simulink model "bat_inv_psm"  (R2025b)
settings: Solver=ode1be  StartTime=0.0  StopTime=simlength  FixedStep=tc  MaxStep=tc
undefined symbols (not defined in the file): b, CTRPIFF_CLIP_RELEASE, dead_time_INV, dead_time_STEPUP, emf_fb_p, emf_fb_p_ccaller_1, emf_fb_p_ccaller_2, emf_p, emf_p_ccaller_1, emf_p_ccaller_2, fPWM_INV, fPWM_STEPUP, g0_161Hz, g1_161Hz, i_grid_neg_eta_lim, i_grid_neg_eta_red_lim, i_grid_neg_xi_lim, i_grid_neg_xi_red_lim, i_grid_pos_eta_lim, i_grid_pos_eta_red_lim, ibez, id_lim, idc_bez, iq_lim, Jm, k_frt_ref, kg, ki_i, ki_ib, ki_vs, ki_w, kp_i, kp_ib, kp_vs, kp_w, kw, l1, l2, Lb, Ld_norm, Lq_norm, Ls_norm, magnitude, motorc_m_scale, number_of_cells, omega_bez, omega_m_bez, omega_m_sim, psi_bez, psi_m, psi_m_norm, Q, q1Kalman, q2Kalman, q3Kalman, rKalman, RLb, rpm_bez, rpm_sim, rpm_torque_curve ... (+17)
libraries: fl_lib x87, nesl_utility x66, simulink x4, singlephase_inductor_with_saturation_lib x2, threephase_inductor_lib x1, ee_lib x1, lithium_ion_cell_lib x1, flexshaft_lib x1, pmsm_uvw_with_harmonics_lib x1
(part 3 of 5)

== system bat_inv_psm/afe_abc_inv_psm_mod1/stepup/switch_2 ==
  Diode : fl_lib/Electrical/Electrical Elements/Diode  Vf=Vgamma V  Ron=Ron Ohm  Goff=1e-8 1/Ohm  i_specify=off  i_priority=None  i=0 A  i_nominal_specify=off  i_nominal_value=1  i_nominal_unit=A  v_specify=off  v_priority=None  v=0 V  v_nominal_specify=off  v_nominal_value=1  v_nominal_unit=V
  Switch : fl_lib/Electrical/Electrical Elements/Switch  R_closed=Ron Ohm  G_open=1e-8 1/Ohm  Threshold=7.5  i_specify=off  i_priority=None  i=0 A  i_nominal_specify=off  i_nominal_value=1  i_nominal_unit=A  v_specify=off  v_priority=None  v=0 V  v_nominal_specify=off  v_nominal_value=1  v_nominal_unit=V
  snubber : fl_lib/Electrical/Electrical Elements/Capacitor  c=Csnubber F  r=Rsnubber Ohm  g=0 1/Ohm  i_specify=off  i_priority=None  i=0 A  i_nominal_specify=off  i_nominal_value=1  i_nominal_unit=A  v_specify=off  v_priority=None  v=0 V  v_nominal_specify=off  v_nominal_value=1  v_nominal_unit=V  vc_specify=off  vc_priority=High  vc=0 V  vc_nominal_specify=off  vc_nominal_value=1  vc_nominal_unit=V
  G : PMIOPort  Side=Left
  C : PMIOPort  Port=2  Side=Left
  E : PMIOPort  Port=3  Side=Right
  connections:
  Switch/RConn2 -- C/RConn1 -- snubber/LConn1 -- Diode/RConn1
  Switch/RConn1 -- G/RConn1
  Switch/LConn1 -- E/RConn1 -- snubber/RConn1 -- Diode/LConn1

== system bat_inv_psm/afe_abc_inv_psm_mod1/stepup_control/idc_ctrl ==
  idc_pu : Inport
  idc_pu_ref : Inport  Port=2
  1/Ti : Gain  Gain=kp_ib  SaturateOnIntegerOverflow=on  OutDataTypeStr=Inherit: Same as input  ParamDataTypeStr=Inherit: Same as input
  Gain : Gain
  Saturation : Saturate  UpperLimit=1  LowerLimit=0
  Sum1 : Sum  Inputs=+++  SaturateOnIntegerOverflow=on
  Sum2 : Sum  Inputs=-+  SaturateOnIntegerOverflow=on
  Sum3 : Sum  Inputs=-+  SaturateOnIntegerOverflow=on
  Unit Delay1 : UnitDelay  SampleTime=ts_stepup  HasFrameUpgradeWarning=on
  Unit Delay4 : UnitDelay  SampleTime=ts_stepup  HasFrameUpgradeWarning=on
  kp : Gain  Gain=ki_ib*ts_stepup  SaturateOnIntegerOverflow=on  OutDataTypeStr=Inherit: Same as input  ParamDataTypeStr=Inherit: Same as input
  m_stepup : Outport
  wires:
  Gain/1 -> Unit Delay1/1
  Saturation/1 -> Sum3/2, Gain/1
  Sum1/1 -> Saturation/1
  Sum2/1 -> 1/Ti/1, kp/1
  idc_pu/1 -> Sum2/1
  idc_pu_ref/1 -> Sum2/2
  Unit Delay4/1 -> Sum1/3
  Sum3/1 -> Unit Delay4/1
  kp/1 -> Sum1/2
  1/Ti/1 -> Sum3/1, Sum1/1
  Unit Delay1/1 -> m_stepup/1

== system bat_inv_psm/afe_abc_inv_psm_mod1/stepup_control/udc_ctrl ==
  udc_pu : Inport
  udc_pu_ref : Inport  Port=2
  1/Ti : Gain  Gain=kp_vs  SaturateOnIntegerOverflow=on  OutDataTypeStr=Inherit: Same as input  ParamDataTypeStr=Inherit: Same as input
  Gain : Gain
  Saturation : Saturate  UpperLimit=1.4  LowerLimit=-1.4
  Sum1 : Sum  Inputs=+++  SaturateOnIntegerOverflow=on
  Sum2 : Sum  Inputs=-+  SaturateOnIntegerOverflow=on
  Sum3 : Sum  Inputs=-+  SaturateOnIntegerOverflow=on
  Unit Delay4 : UnitDelay  SampleTime=ts_stepup  HasFrameUpgradeWarning=on
  kp : Gain  Gain=ki_vs*ts_stepup  SaturateOnIntegerOverflow=on  OutDataTypeStr=Inherit: Same as input  ParamDataTypeStr=Inherit: Same as input
  idc_ref : Outport
  wires:
  1/Ti/1 -> Sum3/1, Sum1/1
  kp/1 -> Sum1/2
  Sum3/1 -> Unit Delay4/1
  Unit Delay4/1 -> Sum1/3
  udc_pu_ref/1 -> Sum2/2
  udc_pu/1 -> Sum2/1
  Sum2/1 -> kp/1, 1/Ti/1
  Sum1/1 -> Saturation/1
  Saturation/1 -> Sum3/2, Gain/1
  Gain/1 -> idc_ref/1

== system bat_inv_psm/battery/battery_system/LithiumIonBattery ==
  Current Sensor : fl_lib/Electrical/Electrical Sensors/Current Sensor
  Electrical Reference1 : fl_lib/Electrical/Electrical Elements/Electrical Reference
  PS-Simulink Converter4 : nesl_utility/PS-Simulink Converter  PhysicalDomain=network_engine_domain  SubClassName=ps_output  LeftPortType=input  RightPortType=output  PseudoPeriodic=off  Frequencies=[]  VectorFormat=1-D array  Unit=1  AffineConversion=off
  PS-Simulink Converter5 : nesl_utility/PS-Simulink Converter  PhysicalDomain=network_engine_domain  SubClassName=ps_output  LeftPortType=input  RightPortType=output  PseudoPeriodic=off  Frequencies=[]  VectorFormat=1-D array  Unit=V  AffineConversion=on
  SOC_estimator : Subsystem  Commented=on
  To Workspace1 : ToWorkspace  VariableName=idc_battery_sim  SampleTime=tc
      settings: MaxDataPoints=Nc
  To Workspace2 : ToWorkspace  VariableName=udc_battery_sim  SampleTime=tc
      settings: MaxDataPoints=Nc
  Unit Delay5 : UnitDelay  SampleTime=ts_stepup  HasFrameUpgradeWarning=on
  Voltage Sensor : fl_lib/Electrical/Electrical Sensors/Voltage Sensor
  ibat/vdc : Scope  NumInputPorts=2
      settings: SampleTime=tc  ActiveDisplayYMinimum=-1320.0904644876443  ActiveDisplayYMaximum=5476.2315205150016  DataLoggingVariableName=ScopeData6
  lithium ion cell analytical ocv : Subsystem
  Uout+ : PMIOPort  Side=Right
  Uout- : PMIOPort  Port=2  Side=Right
  wires:
  PS-Simulink Converter5/1 -> Unit Delay5/1
  PS-Simulink Converter4/1 -> To Workspace1/1, ibat/vdc/1  "i batt"
  Unit Delay5/1 -> To Workspace2/1, [vdc]
  [vdc] -> ibat/vdc/2  "vdc"
  connections:
  Current Sensor/RConn1 -- PS-Simulink Converter4/LConn1
  Uout+/RConn1 -- Current Sensor/RConn2 -- Voltage Sensor/LConn1
  Voltage Sensor/RConn1 -- PS-Simulink Converter5/LConn1
  Voltage Sensor/RConn2 -- Electrical Reference1/LConn1 -- lithium ion cell analytical ocv/RConn2 -- Uout-/RConn1
  lithium ion cell analytical ocv/RConn1 -- Current Sensor/LConn1

== system bat_inv_psm/afe_abc_inv_psm_mod1/inverter/inverter/sv_pwm ==
  ab : Inport
  enable : Inport  Port=2
  Bus Selector : BusSelector  OutputSignals=da,db,dc
  Bus Selector1 : BusSelector  OutputSignals=ua,ub
  C Caller : CCaller  FunctionName=sv_pwm_process_simulink  PortSpecificationStruct="%)30     .    V @   8    (     @         %    \"     4    !     0         %  0 \"0    $    _    07)G3F%M90  4&]R=$YA;64 4V-O<&4     26YD97@     5'EP90      4VEZ90      27-';&]B86P   X    P    !@    @    $          4    (     0    ,    !         !   P!O=70 #@   #     &    \"     0         !0    @    !     P    $         $  # &]U=  .    .     8    (    !          %    \"     $    &     0         0   ...(+2669 chars)"  SampleTime=ts_inv
  Constant : Constant  Value=ts_inv
  Data Type Conversion1 : DataTypeConversion  OutDataTypeStr=double  SaturateOnIntegerOverflow=off  RndMeth=Floor
  Data Type Conversion15 : DataTypeConversion  OutDataTypeStr=single  SaturateOnIntegerOverflow=off  RndMeth=Floor
  Data Type Conversion16 : DataTypeConversion  OutDataTypeStr=single  SaturateOnIntegerOverflow=off  RndMeth=Floor
  Data Type Conversion17 : DataTypeConversion  OutDataTypeStr=uint32  SaturateOnIntegerOverflow=off  RndMeth=Floor
  Data Type Conversion18 : DataTypeConversion  OutDataTypeStr=single  SaturateOnIntegerOverflow=off  RndMeth=Floor
  Data Type Conversion2 : DataTypeConversion  OutDataTypeStr=double  SaturateOnIntegerOverflow=off  RndMeth=Floor
  Data Type Conversion3 : DataTypeConversion  OutDataTypeStr=double  SaturateOnIntegerOverflow=off  RndMeth=Floor
  Zero-Order Hold{,1..3} (4 alike) : ZeroOrderHold  SampleTime=ts_afe
  modulator1 : Subsystem
  firing_gates : Outport
  wires:
  Data Type Conversion1/1 -> modulator1/1(u)  "du"
  Zero-Order Hold/1 -> C Caller/1
  Zero-Order Hold2/1 -> C Caller/3
  Constant/1 -> Data Type Conversion16/1
  Data Type Conversion18/1 -> Zero-Order Hold/1
  enable/1 -> Data Type Conversion17/1
  Data Type Conversion2/1 -> modulator1/2(v)  "dv"
  Data Type Conversion16/1 -> Zero-Order Hold2/1
  Zero-Order Hold1/1 -> C Caller/2
  Data Type Conversion17/1 -> Zero-Order Hold3/1
  Zero-Order Hold3/1 -> C Caller/4
  Data Type Conversion15/1 -> Zero-Order Hold1/1
  C Caller/1 -> Bus Selector/1  "out"
  Data Type Conversion3/1 -> modulator1/3(w)  "dw"
  modulator1/1(cmd_gates) -> firing_gates/1
  ab/1 -> Bus Selector1/1
  Bus Selector1/1 -> Data Type Conversion18/1  "<ua>"
  Bus Selector1/2 -> Data Type Conversion15/1  "<ub>"
  Bus Selector/1 -> Data Type Conversion1/1  "<da>"
  Bus Selector/3 -> Data Type Conversion3/1  "<dc>"
  Bus Selector/2 -> Data Type Conversion2/1  "<db>"

== system bat_inv_psm/afe_abc_inv_psm_mod1/inverter/inverter/switch_1 ==
  Diode : fl_lib/Electrical/Electrical Elements/Diode  Vf=Vgamma V  Ron=Ron Ohm  Goff=1e-8 1/Ohm  i_specify=off  i_priority=None  i=0 A  i_nominal_specify=off  i_nominal_value=1  i_nominal_unit=A  v_specify=off  v_priority=None  v=0 V  v_nominal_specify=off  v_nominal_value=1  v_nominal_unit=V
  Switch : fl_lib/Electrical/Electrical Elements/Switch  R_closed=Ron Ohm  G_open=1e-8 1/Ohm  Threshold=7.5  i_specify=off  i_priority=None  i=0 A  i_nominal_specify=off  i_nominal_value=1  i_nominal_unit=A  v_specify=off  v_priority=None  v=0 V  v_nominal_specify=off  v_nominal_value=1  v_nominal_unit=V
  G : PMIOPort  Side=Left
  C : PMIOPort  Port=2  Side=Left
  E : PMIOPort  Port=3  Side=Right
  connections:
  Switch/RConn2 -- C/RConn1 -- Diode/RConn1
  Switch/RConn1 -- G/RConn1
  Switch/LConn1 -- E/RConn1 -- Diode/LConn1

== system bat_inv_psm/afe_abc_inv_psm_mod1/inverter/inverter/switch_2 ==
  Diode : fl_lib/Electrical/Electrical Elements/Diode  Vf=Vgamma V  Ron=Ron Ohm  Goff=1e-8 1/Ohm  i_specify=off  i_priority=None  i=0 A  i_nominal_specify=off  i_nominal_value=1  i_nominal_unit=A  v_specify=off  v_priority=None  v=0 V  v_nominal_specify=off  v_nominal_value=1  v_nominal_unit=V
  Switch : fl_lib/Electrical/Electrical Elements/Switch  R_closed=Ron Ohm  G_open=1e-8 1/Ohm  Threshold=7.5  i_specify=off  i_priority=None  i=0 A  i_nominal_specify=off  i_nominal_value=1  i_nominal_unit=A  v_specify=off  v_priority=None  v=0 V  v_nominal_specify=off  v_nominal_value=1  v_nominal_unit=V
  G : PMIOPort  Side=Left
  C : PMIOPort  Port=2  Side=Left
  E : PMIOPort  Port=3  Side=Right
  connections:
  Diode/LConn1 -- E/RConn1 -- Switch/LConn1
  Switch/RConn1 -- G/RConn1
  Diode/RConn1 -- C/RConn1 -- Switch/RConn2

== system bat_inv_psm/afe_abc_inv_psm_mod1/inverter/inverter/switch_3 ==
  Diode : fl_lib/Electrical/Electrical Elements/Diode  Vf=Vgamma V  Ron=Ron Ohm  Goff=1e-8 1/Ohm  i_specify=off  i_priority=None  i=0 A  i_nominal_specify=off  i_nominal_value=1  i_nominal_unit=A  v_specify=off  v_priority=None  v=0 V  v_nominal_specify=off  v_nominal_value=1  v_nominal_unit=V
  Switch : fl_lib/Electrical/Electrical Elements/Switch  R_closed=Ron Ohm  G_open=1e-8 1/Ohm  Threshold=7.5  i_specify=off  i_priority=None  i=0 A  i_nominal_specify=off  i_nominal_value=1  i_nominal_unit=A  v_specify=off  v_priority=None  v=0 V  v_nominal_specify=off  v_nominal_value=1  v_nominal_unit=V
  G : PMIOPort  Side=Left
  C : PMIOPort  Port=2  Side=Left
  E : PMIOPort  Port=3  Side=Right
  connections:
  Diode/LConn1 -- E/RConn1 -- Switch/LConn1
  Switch/RConn1 -- G/RConn1
  Diode/RConn1 -- C/RConn1 -- Switch/RConn2

== system bat_inv_psm/afe_abc_inv_psm_mod1/inverter/inverter/switch_4 ==
  Diode : fl_lib/Electrical/Electrical Elements/Diode  Vf=Vgamma V  Ron=Ron Ohm  Goff=1e-8 1/Ohm  i_specify=off  i_priority=None  i=0 A  i_nominal_specify=off  i_nominal_value=1  i_nominal_unit=A  v_specify=off  v_priority=None  v=0 V  v_nominal_specify=off  v_nominal_value=1  v_nominal_unit=V
  Switch : fl_lib/Electrical/Electrical Elements/Switch  R_closed=Ron Ohm  G_open=1e-8 1/Ohm  Threshold=7.5  i_specify=off  i_priority=None  i=0 A  i_nominal_specify=off  i_nominal_value=1  i_nominal_unit=A  v_specify=off  v_priority=None  v=0 V  v_nominal_specify=off  v_nominal_value=1  v_nominal_unit=V
  G : PMIOPort  Side=Left
  C : PMIOPort  Port=2  Side=Left
  E : PMIOPort  Port=3  Side=Right
  connections:
  Switch/RConn2 -- C/RConn1 -- Diode/RConn1
  Switch/RConn1 -- G/RConn1
  Switch/LConn1 -- E/RConn1 -- Diode/LConn1

== system bat_inv_psm/afe_abc_inv_psm_mod1/inverter/inverter/switch_5 ==
  Diode : fl_lib/Electrical/Electrical Elements/Diode  Vf=Vgamma V  Ron=Ron Ohm  Goff=1e-8 1/Ohm  i_specify=off  i_priority=None  i=0 A  i_nominal_specify=off  i_nominal_value=1  i_nominal_unit=A  v_specify=off  v_priority=None  v=0 V  v_nominal_specify=off  v_nominal_value=1  v_nominal_unit=V
  Switch : fl_lib/Electrical/Electrical Elements/Switch  R_closed=Ron Ohm  G_open=1e-8 1/Ohm  Threshold=7.5  i_specify=off  i_priority=None  i=0 A  i_nominal_specify=off  i_nominal_value=1  i_nominal_unit=A  v_specify=off  v_priority=None  v=0 V  v_nominal_specify=off  v_nominal_value=1  v_nominal_unit=V
  G : PMIOPort  Side=Left
  C : PMIOPort  Port=2  Side=Left
  E : PMIOPort  Port=3  Side=Right
  connections:
  Diode/LConn1 -- E/RConn1 -- Switch/LConn1
  Switch/RConn1 -- G/RConn1
  Diode/RConn1 -- C/RConn1 -- Switch/RConn2

== system bat_inv_psm/afe_abc_inv_psm_mod1/inverter/inverter/switch_6 ==
  Diode : fl_lib/Electrical/Electrical Elements/Diode  Vf=Vgamma V  Ron=Ron Ohm  Goff=1e-8 1/Ohm  i_specify=off  i_priority=None  i=0 A  i_nominal_specify=off  i_nominal_value=1  i_nominal_unit=A  v_specify=off  v_priority=None  v=0 V  v_nominal_specify=off  v_nominal_value=1  v_nominal_unit=V
  Switch : fl_lib/Electrical/Electrical Elements/Switch  R_closed=Ron Ohm  G_open=1e-8 1/Ohm  Threshold=7.5  i_specify=off  i_priority=None  i=0 A  i_nominal_specify=off  i_nominal_value=1  i_nominal_unit=A  v_specify=off  v_priority=None  v=0 V  v_nominal_specify=off  v_nominal_value=1  v_nominal_unit=V
  G : PMIOPort  Side=Left
  C : PMIOPort  Port=2  Side=Left
  E : PMIOPort  Port=3  Side=Right
  connections:
  Switch/RConn2 -- C/RConn1 -- Diode/RConn1
  Switch/RConn1 -- G/RConn1
  Switch/LConn1 -- E/RConn1 -- Diode/LConn1

== system bat_inv_psm/afe_abc_inv_psm_mod1/inverter_control/current_ctrl/bemf_observer ==
  ialpha_pu : Inport
  ibeta_pu : Inport  Port=2
  ualpha_pu : Inport  Port=3
  ubeta_pu : Inport  Port=4
  BEMF Observer simulink/Ccaller : Scope  NumInputPorts=2
      settings: SampleTime=tc  ActiveDisplayYMinimum=-1.2577905803918839  ActiveDisplayYMaximum=1.2568866163492203
  Mux : Mux  Inputs=3
  Mux1 : Mux  Inputs=3
  Variant Source : VariantSource  VariantControls={use_observer_from_simulink_module_1 == 1, use_observer_from_ccaller_module_1 == 1}
  Variant Source1 : VariantSource  VariantControls={use_observer_from_simulink_module_1 == 1, use_observer_from_ccaller_module_1 == 1}
  bemf_observer : Subsystem
  bemf_observer_ccaller : Subsystem
  double_integrator_observer : Subsystem
  phase_fault : Subsystem
  tag scope: omega_hat_pu=global, theta_hat=global
  wires:
  ialpha_pu/1 -> bemf_observer/1(ialpha_pu), bemf_observer_ccaller/1(ialpha_pu)
  ibeta_pu/1 -> bemf_observer/2(ibeta_pu), bemf_observer_ccaller/2(ibeta_pu)
  Mux/1 -> BEMF Observer simulink/Ccaller/1
  Mux1/1 -> BEMF Observer simulink/Ccaller/2
  double_integrator_observer/1(omega_pu_hat) -> Mux/3  "omega_pu_encoder"
  ualpha_pu/1 -> bemf_observer/3(ualpha_pu), bemf_observer_ccaller/3(ualpha_pu)
  ubeta_pu/1 -> bemf_observer/4(ubeta_pu), bemf_observer_ccaller/4(ubeta_pu)
  double_integrator_observer/2(theta_hat) -> Mux1/3  "theta_hat_encoder"
  [theta_elec_pmsm] -> phase_fault/1(theta_pmsm)  "theta_pmsm"
  phase_fault/1(theta) -> double_integrator_observer/1(theta)
  bemf_observer/1(omega_pu) -> Mux/1, Variant Source/1  "omega_pu"
  bemf_observer_ccaller/2(theta_hat) -> Mux1/2, Variant Source1/2  "theta_hat_code"
  bemf_observer_ccaller/1(omega_pu) -> Mux/2, Variant Source/2  "omega_pu_code"
  bemf_observer/2(theta_hat) -> Variant Source1/1, Mux1/1  "theta_hat"
  Variant Source1/1 -> [theta_hat]
  Variant Source/1 -> [omega_hat_pu]

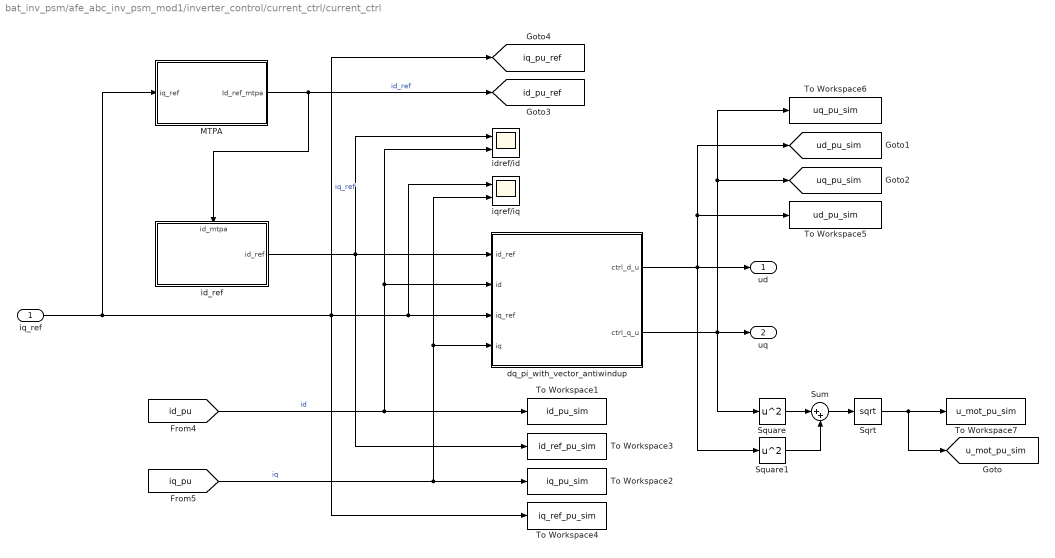
== system bat_inv_psm/afe_abc_inv_psm_mod1/inverter_control/current_ctrl/current_ctrl ==
  iq_ref : Inport
  MTPA : Subsystem
  Sqrt : Sqrt
  Square : Math  Operator=square
  Square1 : Math  Operator=square
  Sum : Sum  Inputs=|++
  To Workspace1 : ToWorkspace  VariableName=id_pu_sim  SampleTime=ts_inv
      settings: MaxDataPoints=Ns_inv
  To Workspace2 : ToWorkspace  VariableName=iq_pu_sim  SampleTime=ts_inv
      settings: MaxDataPoints=Ns_inv
  To Workspace3 : ToWorkspace  VariableName=id_ref_pu_sim  SampleTime=ts_inv
      settings: MaxDataPoints=Ns_inv
  To Workspace4 : ToWorkspace  VariableName=iq_ref_pu_sim  SampleTime=ts_inv
      settings: MaxDataPoints=Ns_inv
  To Workspace5 : ToWorkspace  VariableName=ud_pu_sim  SampleTime=ts_inv
      settings: MaxDataPoints=Ns_inv
  To Workspace6 : ToWorkspace  VariableName=uq_pu_sim  SampleTime=ts_inv
      settings: MaxDataPoints=Ns_inv
  To Workspace7 : ToWorkspace  VariableName=u_mot_pu_sim  SampleTime=ts_inv
      settings: MaxDataPoints=Ns_inv
  dq_pi_with_vector_antiwindup : Subsystem
  id_ref : Subsystem
      settings: PortSchema="{\"entries\":[{\"content\":{\"sides\":[{\"content\":{},\"type\":\"ConnectorPlacement.EquallySpacedRectSide\",\"uuid\":\"42af5d69-f0eb-42c6-9e03-28c1d0757323\"},{\"content\":{\"connectorIds\":[\"Out1\"],\"side\":\"RIGHT\"},\"type\":\"ConnectorPlacement.EquallySpacedRectSide\",\"uuid\":\"dd68a9f9-d15f-4e57-9d9e-130889a7b90c\"},{\"content\":{\"connectorIds\":[\"In1\"],\"side\":\"TOP\"},\"type\":\"ConnectorPlacement.EquallySpacedRectSide\",\"uuid\":\"68c797a2-8439-4b8d-8368-b7485adf0676\"}]},\"type\":\"ConnectorPlacement.EquallySpacedConnector\",\"uuid\":\"693c5f1c-0580-4626-8f13-b27865dfb3ac\"}],\"packageUris\":[\"http://schema.mathworks.com/mf0/Connector/R2020b\"],\"version\":\"1.0\"}"
  idref/id : Scope  NumInputPorts=2
      settings: SampleTime=tc  ActiveDisplayYMinimum=-0.5383825399353187  ActiveDisplayYMaximum=0.059820282309629005
  iqref/iq : Scope  NumInputPorts=2
      settings: SampleTime=tc  ActiveDisplayYMinimum=-1.1641617765003931  ActiveDisplayYMaximum=0.12935130850004364  DataLoggingVariableName=ScopeData2
  ud : Outport
  uq : Outport  Port=2
  tag scope: id_pu_ref=global, iq_pu_ref=global, u_mot_pu_sim=global, ud_pu_sim=global, uq_pu_sim=global
  wires:
  [iq_pu] -> To Workspace2/1, iqref/iq/2, dq_pi_with_vector_antiwindup/4(iq)  "iq"
  [id_pu] -> To Workspace1/1, idref/id/2, dq_pi_with_vector_antiwindup/2(id)  "id"
  MTPA/1(Id_ref_mtpa) -> id_ref/1(id_mtpa), [id_pu_ref]  "id_ref"
  iq_ref/1 -> MTPA/1(iq_ref), To Workspace4/1, iqref/iq/1, dq_pi_with_vector_antiwindup/3(iq_ref), [iq_pu_ref]  "iq_ref"
  dq_pi_with_vector_antiwindup/1(ctrl_d_u) -> To Workspace5/1, [ud_pu_sim], Square1/1, ud/1
  dq_pi_with_vector_antiwindup/2(ctrl_q_u) -> [uq_pu_sim], To Workspace6/1, Square/1, uq/1
  Square/1 -> Sum/1
  Sum/1 -> Sqrt/1
  Square1/1 -> Sum/2
  Sqrt/1 -> [u_mot_pu_sim], To Workspace7/1
  id_ref/1(id_ref) -> To Workspace3/1, dq_pi_with_vector_antiwindup/1(id_ref), idref/id/1

== system bat_inv_psm/afe_abc_inv_psm_mod1/inverter_control/current_ctrl/current_transformation ==
  u : Inport
  v : Inport  Port=2
  w : Inport  Port=3
  To Workspace2 : ToWorkspace  VariableName=ialpha_pu_sim  SampleTime=ts_inv
      settings: MaxDataPoints=Ns_inv
  To Workspace3 : ToWorkspace  VariableName=ibeta_pu_sim  SampleTime=ts_inv
      settings: MaxDataPoints=Ns_inv
  alphabeta2dq : MATLAB Function  TreatAsAtomicUnit=on  SystemSampleTime=ts_inv
  uvw2alphabeta : MATLAB Function  TreatAsAtomicUnit=on  SystemSampleTime=ts_inv
  tag scope: ialpha_pu=global, ibeta_pu=global, id_pu=global, iq_pu=global
  wires:
  w/1 -> uvw2alphabeta/3(w)
  alphabeta2dq/2(q) -> [iq_pu]  "iq_pu"
  alphabeta2dq/1(d) -> [id_pu]  "id_pu"
  v/1 -> uvw2alphabeta/2(v)
  uvw2alphabeta/2(beta) -> To Workspace3/1, [ibeta_pu], alphabeta2dq/2(beta)  "ibeta_pu"
  uvw2alphabeta/1(alpha) -> To Workspace2/1, [ialpha_pu], alphabeta2dq/1(alpha)  "ialpha_pu"
  [theta_hat] -> alphabeta2dq/3(gamma)
  u/1 -> uvw2alphabeta/1(u)

== system bat_inv_psm/afe_abc_inv_psm_mod1/inverter_control/current_ctrl/sample_hold_normalization ==
  iu : Inport
  iv : Inport  Port=2
  iw : Inport  Port=3
  Gain : Gain  Gain=1/ibez
  Gain1 : Gain  Gain=1/ibez
  Gain2 : Gain  Gain=1/ibez
  Quantizer : Quantizer  QuantizationInterval=adc_quantization
  Quantizer1 : Quantizer  QuantizationInterval=adc_quantization
  Quantizer2 : Quantizer  QuantizationInterval=adc_quantization
  Unit Delay : UnitDelay  SampleTime=ts_inv  HasFrameUpgradeWarning=on
  Unit Delay1 : UnitDelay  SampleTime=ts_inv  HasFrameUpgradeWarning=on
  Unit Delay4 : UnitDelay  SampleTime=ts_inv  HasFrameUpgradeWarning=on
  Zero-Order Hold : ZeroOrderHold  SampleTime=ts_inv
  Zero-Order Hold1 : ZeroOrderHold  SampleTime=ts_inv
  Zero-Order Hold2 : ZeroOrderHold  SampleTime=ts_inv
  iu_pu : Outport
  iv_pu : Outport  Port=2
  iw_pu : Outport  Port=3
  wires:
  iu/1 -> Gain/1
  Zero-Order Hold1/1 -> Unit Delay1/1
  Zero-Order Hold2/1 -> Unit Delay4/1
  Zero-Order Hold/1 -> Unit Delay/1
  Unit Delay4/1 -> iw_pu/1
  Unit Delay1/1 -> iv_pu/1
  Unit Delay/1 -> iu_pu/1
  iw/1 -> Gain2/1
  iv/1 -> Gain1/1
  Gain2/1 -> Quantizer2/1
  Gain1/1 -> Quantizer1/1
  Gain/1 -> Quantizer/1
  Quantizer/1 -> Zero-Order Hold/1
  Quantizer1/1 -> Zero-Order Hold1/1
  Quantizer2/1 -> Zero-Order Hold2/1

== system bat_inv_psm/afe_abc_inv_psm_mod1/stepup/dclink_measure/R_derating ==
  Step : Step  After=107.4e3/2  SampleTime=0
  Step1 : Step  Time=1.1  After=-107.4e3/2  SampleTime=0
  Sum : Sum  Inputs=|++
  DR : Outport
  wires:
  Step1/1 -> Sum/2
  Step/1 -> Sum/1
  Sum/1 -> DR/1

== system bat_inv_psm/afe_abc_inv_psm_mod1/stepup/pwm/PWM generator 1 ==
  m_index : Inport
  phase : Inport  Port=2
  Clock : Clock
  Constant : Constant  Value=dead_time*f
  Constant1 : Constant  Value=polarity
  Constant2 : Constant  Value=1/f
  Constant4 : Constant
  Data Type Conversion1 : DataTypeConversion
  Data Type Conversion2 : DataTypeConversion
  Gain4 : Gain  Gain=1/2
  Gain5 : Gain  Gain=1/(pi/2)
  Hit Crossing : HitCross  ShowOutputPort=off
  Hit Crossing1 : HitCross  ShowOutputPort=off
  MATLAB Function : MATLAB Function  TreatAsAtomicUnit=on
  Relational Operator1 : RelationalOperator  Operator=<=  InputSameDT=off
  Relational Operator2 : RelationalOperator  Operator=<=  InputSameDT=off
  Relay : Relay  OnOutputValue=pos_cmd_gate  OffOutputValue=neg_cmd_gate
  Relay1 : Relay  OnOutputValue=pos_cmd_gate  OffOutputValue=neg_cmd_gate
  Saturation1 : Saturate  UpperLimit=m_up  LowerLimit=m_low
  Sum : Sum  Inputs=|++  SaturateOnIntegerOverflow=on
  Sum1 : Sum  Inputs=-+|  SaturateOnIntegerOverflow=on
  Sum3 : Sum  Inputs=|++
  Switch : Switch  Criteria=u2 > Threshold  SaturateOnIntegerOverflow=off  InputSameDT=off
  Switch1 : Switch  Criteria=u2 > Threshold  SaturateOnIntegerOverflow=off  InputSameDT=off
  m1 : Outport
  m2 : Outport  Port=2
  wires:
  Relational Operator1/1 -> Data Type Conversion1/1
  m_index/1 -> Saturation1/1
  Relational Operator2/1 -> Data Type Conversion2/1
  Data Type Conversion2/1 -> Switch/1, Switch1/3, Hit Crossing1/1
  Constant/1 -> Sum/2, Sum1/1
  Saturation1/1 -> Sum/1, Sum1/2
  Sum/1 -> Relational Operator1/1
  Sum1/1 -> Relational Operator2/2
  Gain4/1 -> Relational Operator2/1, Relational Operator1/2
  Data Type Conversion1/1 -> Hit Crossing/1, Switch/3, Switch1/1
  Switch/1 -> Relay/1
  Clock/1 -> MATLAB Function/1(t)
  Constant2/1 -> MATLAB Function/3(period)
  phase/1 -> MATLAB Function/2(phase)
  MATLAB Function/1(y) -> Gain5/1
  Gain5/1 -> Sum3/1
  Sum3/1 -> Gain4/1
  Constant4/1 -> Sum3/2
  Relay/1 -> m2/1
  Constant1/1 -> Switch1/2, Switch/2
  Switch1/1 -> Relay1/1
  Relay1/1 -> m1/1

== system bat_inv_psm/battery/battery_system/LithiumIonBattery/SOC_estimator ==
  Kalman_observer : Subsystem
  SOC*/SOC : Scope  Commented=on  NumInputPorts=2
      settings: SampleTime=tsample  ActiveDisplayYMinimum=-0.16149  ActiveDisplayYMaximum=0.90685
  Selector1 : Selector  InputPortWidth=3  IndexOptions=Index vector (dialog)  Indices=3  OutputSizes=1
  h_hat/h : Scope  Commented=on  NumInputPorts=2
      settings: SampleTime=tsample  ActiveDisplayYMinimum=-0.13002  ActiveDisplayYMaximum=0.15534  DataLoggingVariableName=ScopeData2
  i_out/v_out : Scope  Commented=on  NumInputPorts=2
      settings: SampleTime=tsample  ActiveDisplayYMinimum=-467.64425  ActiveDisplayYMaximum=280.87629  DataLoggingVariableName=ScopeData3
  soc/iout : Scope  Commented=on  NumInputPorts=2
      settings: SampleTime=tsample  ActiveDisplayYMinimum=0.19925  ActiveDisplayYMaximum=0.20008  DataLoggingVariableName=ScopeData4
  wires:
  Kalman_observer/2(SOC) -> SOC*/SOC/2
  Kalman_observer/1(x(k+1|k)) -> Selector1/1
  [im] -> i_out/v_out/1  "im+noise"
  [h] -> h_hat/h/2
  [SOC] -> soc/iout/1, SOC*/SOC/1
  Selector1/1 -> h_hat/h/1  "h_hat(z)"
  [vout] -> Kalman_observer/1(vout(k)), i_out/v_out/2
  [icell] -> soc/iout/2

== system bat_inv_psm/battery/battery_system/LithiumIonBattery/lithium ion cell analytical ocv ==
  Current Sensor : fl_lib/Electrical/Electrical Sensors/Current Sensor
  Electrical Reference : fl_lib/Electrical/Electrical Elements/Electrical Reference
  PS Constant : fl_lib/Physical Signals/Sources/PS Constant  constant=298.15 K
  PS-Simulink Converter{,1..4} (5 alike) : nesl_utility/PS-Simulink Converter  PhysicalDomain=network_engine_domain  SubClassName=ps_output  LeftPortType=input  RightPortType=output  PseudoPeriodic=off  Frequencies=[]  VectorFormat=1-D array  Unit=inherit  AffineConversion=off
  Voltage Sensor : fl_lib/Electrical/Electrical Sensors/Voltage Sensor
  lithium-ion battery with analytical OCV : lithium_ion_cell_lib/lithium-ion Cell with analytical OCV  Qcell=Q hr*A  N=number_of_cells  E_1=E1 V  E0=E0 V  E1=E1 V  E2=E2 V  E3=E3 V  Elog=Elog V  R0=R0 Ohm  R1=R1 Ohm  C1=C1 F  M=M V  alpha=alpha  u_specify=off  u_priority=High  u=Vdc V  u_nominal_specify=off  u_nominal_unit=V  u_nominal_value=1  u_ocv_specify=off  u_ocv_priority=High  u_ocv=Vdc V  u_ocv_nominal_specify=off  u_ocv_nominal_unit=V  u_ocv_nominal_value=1  icell_specify=off  icell_priority=None  icell=0 A  icell_nominal_specify=off  icell_nominal_unit=A  icell_nominal_value=1  i_r1_specify=off  i_r1_priority=None  i_r1=0 A  i_r1_nominal_specify=off  i_r1_nominal_unit=A  i_r1_nominal_value=1  z_specify=on  z_priority=High  z=soc_init  z_nominal_specify=off  z_nominal_unit=1  z_nominal_value=1  h_specify=off  h_priority=High  h=0  h_nominal_specify=off  h_nominal_unit=1  h_nominal_value=1
      settings: InternalSimscapePortConfiguration="{\"Bottom\":[],\"Left\":[{\"id\":\"T\",\"label\":\"T\",\"type\":\"input\"}],\"Right\":[{\"id\":\"u_p\",\"label\":\"u+\",\"type\":\"foundation.electrical.electrical\"},{\"id\":\"u_n\",\"label\":\"u-\",\"type\":\"foundation.electrical.electrical\"},{\"id\":\"z_out\",\"label\":\"SOC\",\"type\":\"output\"},{\"id\":\"i_r1_out\",\"label\":\"i_r1\",\"type\":\"output\"},{\"id\":\"h_out\",\"label\":\"hysteresis\",\"type\":\"output\"}],\"Top\":[]}"
  white_noise : Subsystem
  U+ : PMIOPort  Side=Right
  U- : PMIOPort  Port=2  Side=Right
  tag scope: SOC=global, h=global, icell=global, im=global, vout=global
  wires:
  PS-Simulink Converter/1 -> [vout]  "vout(k)"
  PS-Simulink Converter1/1 -> white_noise/1(in)  "i(k)"
  white_noise/1(out) -> [im]
  PS-Simulink Converter4/1 -> [h]  "h(t)"
  PS-Simulink Converter2/1 -> [icell]  "icell"
  PS-Simulink Converter3/1 -> [SOC]  "SOC*"
  connections:
  lithium-ion battery with analytical OCV/LConn1 -- PS Constant/RConn1
  PS-Simulink Converter/LConn1 -- Voltage Sensor/RConn1
  Current Sensor/RConn2 -- Voltage Sensor/LConn1 -- U+/RConn1
  Electrical Reference/LConn1 -- Voltage Sensor/RConn2 -- U-/RConn1 -- lithium-ion battery with analytical OCV/RConn2
  Current Sensor/RConn1 -- PS-Simulink Converter1/LConn1
  lithium-ion battery with analytical OCV/RConn1 -- Current Sensor/LConn1
  lithium-ion battery with analytical OCV/RConn3 -- PS-Simulink Converter3/LConn1
  lithium-ion battery with analytical OCV/RConn4 -- PS-Simulink Converter2/LConn1
  lithium-ion battery with analytical OCV/RConn5 -- PS-Simulink Converter4/LConn1

== system bat_inv_psm/afe_abc_inv_psm_mod1/inverter/inverter/sv_pwm/modulator1 ==
  u : Inport
  v : Inport  Port=2
  w : Inport  Port=3
  phase : Inport  Port=4
  Bus Creator3 : BusCreator  Inputs=6
  PWM generator 1 : Subsystem  mask{f=fPWM_INV, m_up=0.98, m_low=0.02, dead_time=dead_time_INV, pos_cmd_gate=15, neg_cmd_gate=-10, polarity=1}
      mask prompts: f "Frequency (Hz)"; m_up "Max Input Modulation Value"; m_low "Min Input Modulation Value"; dead_time "Dead Time (s)"; pos_cmd_gate "Positive Gate Voltage (V)"; neg_cmd_gate "Negative Gate Voltage (V)"; polarity "Polarity (pu)"
  PWM generator 2 : Subsystem  mask{f=fPWM_INV, m_up=0.98, m_low=0.02, dead_time=dead_time_INV, pos_cmd_gate=15, neg_cmd_gate=-10, polarity=1}
      mask prompts: f "Frequency (Hz)"; m_up "Max Input Modulation Value"; m_low "Min Input Modulation Value"; dead_time "Dead Time (s)"; pos_cmd_gate "Positive Gate Voltage (V)"; neg_cmd_gate "Negative Gate Voltage (V)"; polarity "Polarity (pu)"
  PWM generator 3 : Subsystem  mask{f=fPWM_INV, m_up=0.98, m_low=0.02, dead_time=dead_time_INV, pos_cmd_gate=15, neg_cmd_gate=-10, polarity=1}
      mask prompts: f "Frequency (Hz)"; m_up "Max Input Modulation Value"; m_low "Min Input Modulation Value"; dead_time "Dead Time (s)"; pos_cmd_gate "Positive Gate Voltage (V)"; neg_cmd_gate "Negative Gate Voltage (V)"; polarity "Polarity (pu)"
  cmd_gates : Outport
  wires:
  u/1 -> PWM generator 1/1(m_index)
  w/1 -> PWM generator 3/1(m_index)
  v/1 -> PWM generator 2/1(m_index)
  phase/1 -> PWM generator 3/2(phase), PWM generator 2/2(phase), PWM generator 1/2(phase)
  PWM generator 1/2(m2) -> Bus Creator3/2  "pwm_inverter_phase_u_bottom"
  PWM generator 3/1(m1) -> Bus Creator3/5  "pwm_inverter_phase_w_top"
  PWM generator 2/1(m1) -> Bus Creator3/3  "pwm_inverter_phase_v_top"
  PWM generator 2/2(m2) -> Bus Creator3/4  "pwm_inverter_phase_v_bottom"
  PWM generator 3/2(m2) -> Bus Creator3/6  "pwm_inverter_phase_w_bottom"
  PWM generator 1/1(m1) -> Bus Creator3/1  "pwm_inverter_phase_u_top"
  Bus Creator3/1 -> cmd_gates/1

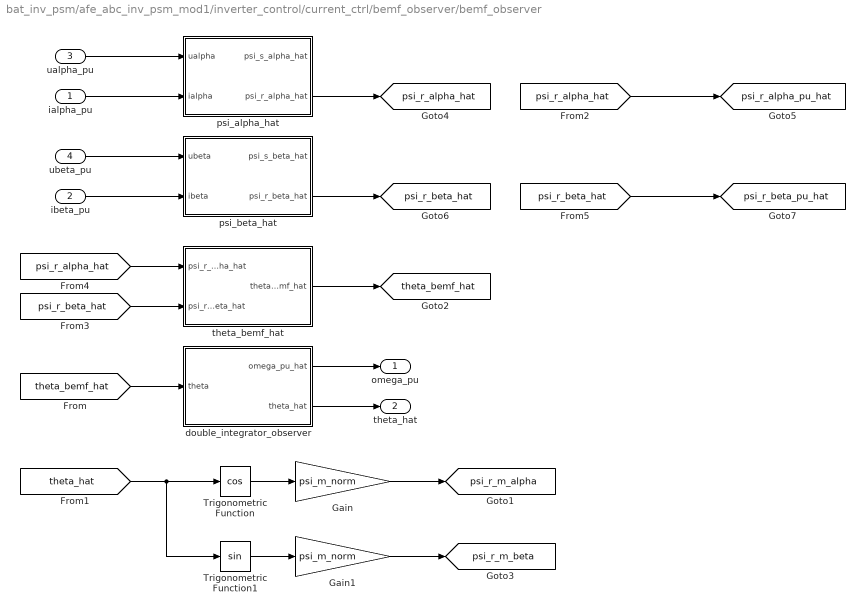
== system bat_inv_psm/afe_abc_inv_psm_mod1/inverter_control/current_ctrl/bemf_observer/bemf_observer ==
  ialpha_pu : Inport
  ibeta_pu : Inport  Port=2
  ualpha_pu : Inport  Port=3
  ubeta_pu : Inport  Port=4
  Gain : Gain  Gain=psi_m_norm
  Gain1 : Gain  Gain=psi_m_norm
  Trigonometric Function : Trigonometry  Operator=cos
  Trigonometric Function1 : Trigonometry
  double_integrator_observer : Subsystem
  psi_alpha_hat : Subsystem
  psi_beta_hat : Subsystem
  theta_bemf_hat : Subsystem
  omega_pu : Outport
  theta_hat : Outport  Port=2
  tag scope: psi_r_alpha_hat=global, psi_r_alpha_pu_hat=global, psi_r_beta_hat=global, psi_r_beta_pu_hat=global, psi_r_m_alpha=global, psi_r_m_beta=global, theta_bemf_hat=global
  wires:
  Trigonometric Function/1 -> Gain/1
  Trigonometric Function1/1 -> Gain1/1
  ialpha_pu/1 -> psi_alpha_hat/2(ialpha)
  ibeta_pu/1 -> psi_beta_hat/2(ibeta)
  psi_alpha_hat/2(psi_r_alpha_hat) -> [psi_r_alpha_hat]
  psi_beta_hat/2(psi_r_beta_hat) -> [psi_r_beta_hat]
  [psi_r_alpha_hat] -> theta_bemf_hat/1(psi_r_alpha_hat)
  [psi_r_beta_hat] -> theta_bemf_hat/2(psi_r_beta_hat)
  ualpha_pu/1 -> psi_alpha_hat/1(ualpha)
  ubeta_pu/1 -> psi_beta_hat/1(ubeta)
  [theta_hat] -> Trigonometric Function/1, Trigonometric Function1/1
  Gain/1 -> [psi_r_m_alpha]
  Gain1/1 -> [psi_r_m_beta]
  theta_bemf_hat/1(theta_emf_hat) -> [theta_bemf_hat]
  [theta_bemf_hat] -> double_integrator_observer/1(theta)
  double_integrator_observer/1(omega_pu_hat) -> omega_pu/1
  double_integrator_observer/2(theta_hat) -> theta_hat/1
  [psi_r_alpha_hat] -> [psi_r_alpha_pu_hat]
  [psi_r_beta_hat] -> [psi_r_beta_pu_hat]
